simulink model "Prj_1_E"  (R2023a)
settings: Solver=VariableStepAuto  StartTime=0.0  StopTime=600  RelTol=1e-3
model workspace (MAT data in the model file):
  C_0 = 0.015
  M_veh = 1746
  g = 9.8
values from neighbouring files (symbols this model uses):
  A_F = params.FrontalArea_m2_    [Old_Init.m]    (also in init.m; old_script.m)
  C_D = params.Cd    [init.m]
  eta_ess = 0.8    [Old_Init.m]    (also in init.m; old_script.m)
  G_diff = 0.268    [Old_Init.m]    (also in init.m; old_script.m)
  G_elec = 1    [Old_Init.m]    (also in init.m; old_script.m)
  r_wheel = params.WheelRadius_meters_    [init.m]
  rho = params.AirDensity    [init.m]
  SOC_init = 0.5    [Old_Init.m]    (also in init.m; loadVehicleParams.m; old_script.m)
undefined symbols (not defined in the file or in its folder): E_ess_max, eng_map, g_per_hr_to_gal_per_s, m_to_mi, mi_per_hr_to_m_per_s, param, us06
libraries: visionstatistics x1
settings Model: Creator=manuel  LastModifiedBy=Manuel
settings SolverCC: ZeroCrossAlgorithm=Adaptive  AlgebraicLoopSolver=TrustRegion
settings DebuggingCC: MaskedZcDiagnostic=none  IgnoredZcDiagnostic=none  UnconnectedInputMsg=warning  UnconnectedOutputMsg=warning  UnconnectedLineMsg=warning
settings ModelReferenceCC: EnableRefExpFcnMdlSchedulingChecks=on

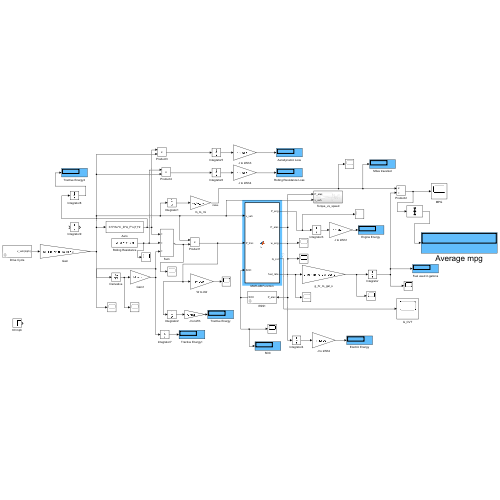
[thumbnail: Simulink's stored preview of the top-level diagram]
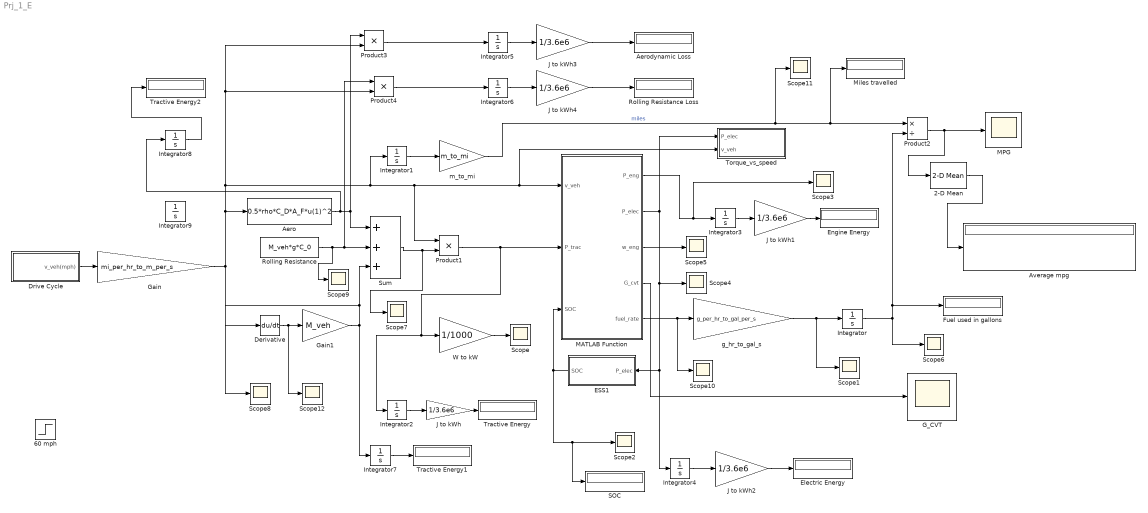
== system Prj_1_E ==
  2-D Mean : visionstatistics/2-D Mean  run=off  reset_popup=None  directionMode=Entire input  dimension=1  treatSBRowAsCol=on  outputLastDataTypeStr=Inherit: Same as accumulator  accumMode=Binary point scaling  accumWordLength=32  accumFracLength=0  accumLastDataTypeStr=fixdt([],32,0)  roiEnable=off  roiType=Rectangles  roiPortion=Entire ROI  roiOutput=Individual statistics for each ROI  roiFlag=off  roundingMode=Floor  overflowMode=off  accumDataTypeStr=fixdt([],32,0)  outputDataTypeStr=Inherit: Same as accumulator  outputMin=[]  outputMax=[]
  60 mph : Step  Before=60  After=60  SampleTime=0
  Aero : Fcn  Expr=0.5*rho*C_D*A_F*u(1)^2
  Aerodynamic Loss : Display
  Average mpg : Display
      settings: Decimation=3
  Derivative : Derivative
  Drive Cycle : Subsystem  mask{schedule=us06}
      mask prompts: schedule "drive schedule"
      mask init:
      | N=length(schedule(:,1))
  ESS1 : Subsystem  mask{E_max=E_ess_max, eta_ess=eta_ess}
      mask prompts: E_max "Maximum energy, J"; eta_ess "round-trip efficiency"
  Electric Energy : Display
  "Engine Energy " : Display
  Fuel used in gallons : Display
  G_CVT : Scope
  Gain : Gain  Gain=mi_per_hr_to_m_per_s
  Gain1 : Gain  Gain=M_veh
  Integrator{,1..9} (10 alike) : Integrator
  J to kWh{,1..4} (5 alike) : Gain  Gain=1/3.6e6
  MATLAB Function : MATLAB Function  TreatAsAtomicUnit=on
  MPG : Scope
  Miles travelled : Display
  Product1 : Product
  Product2 : Product  Inputs=*/
  Product3 : Product
  Product4 : Product
  Rolling Resistance : Constant  Value=M_veh*g*C_0
  Rolling Resistance Loss : Display
  SOC : Display
  Scope{,1..12} (13 alike) : Scope
  Sum : Sum  Inputs=+++
  Torque_vs_speed : Subsystem
  Tractive Energy : Display
  Tractive Energy1 : Display
  Tractive Energy2 : Display
  W to kW : Gain  Gain=1/1000
  g_hr_to_gal_s : Gain  Gain=g_per_hr_to_gal_per_s
  m_to_mi : Gain  Gain=m_to_mi
  wires:
  Aero/1 -> Integrator8/1, Sum/1, Product3/1
  Rolling Resistance/1 -> Scope9/1, Product4/1, Sum/2
  Sum/1 -> Scope7/1, Product1/2
  MATLAB Function/2(P_elec) -> Torque_vs_speed/1(P_elec), Scope4/1, Integrator4/1, ESS1/1(P_elec)
  Gain/1 -> Aero/1, Product1/1, Torque_vs_speed/2(v_veh), MATLAB Function/1(v_veh), Integrator1/1, Product4/2, Product3/2, Derivative/1
  g_hr_to_gal_s/1 -> Integrator/1, Scope1/1
  Integrator1/1 -> m_to_mi/1
  MATLAB Function/1(P_eng) -> Integrator3/1, Scope3/1
  MATLAB Function/3(w_eng) -> Scope5/1
  m_to_mi/1 -> Product2/1, Miles travelled/1, Scope11/1  "miles"
  MATLAB Function/4(G_cvt) -> G_CVT/1
  W to kW/1 -> Scope/1
  Integrator/1 -> Product2/2, Fuel used in gallons/1, Scope6/1
  ESS1/1(SOC) -> SOC/1, Scope2/1, MATLAB Function/3(SOC)
  Product1/1 -> W to kW/1, Integrator2/1, MATLAB Function/2(P_trac)
  Integrator2/1 -> J to kWh/1
  J to kWh/1 -> Tractive Energy/1
  Integrator3/1 -> J to kWh1/1
  J to kWh1/1 -> "Engine Energy "/1
  Integrator4/1 -> J to kWh2/1
  J to kWh2/1 -> Electric Energy/1
  Integrator5/1 -> J to kWh3/1
  J to kWh3/1 -> Aerodynamic Loss/1
  Product3/1 -> Integrator5/1
  Product4/1 -> Integrator6/1
  Integrator6/1 -> J to kWh4/1
  J to kWh4/1 -> Rolling Resistance Loss/1
  Product2/1 -> 2-D Mean/1, MPG/1
  2-D Mean/1 -> Average mpg/1
  MATLAB Function/5(fuel_rate) -> Scope10/1, g_hr_to_gal_s/1
  Drive Cycle/1(v_veh(mph)) -> Gain/1
  Derivative/1 -> Scope12/1, Gain1/1
  Gain1/1 -> Integrator7/1, Scope8/1, Sum/3
  Integrator7/1 -> Tractive Energy1/1
  Integrator8/1 -> Tractive Energy2/1

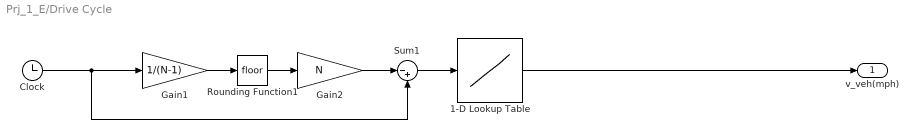
== system Prj_1_E/Drive Cycle ==
  1-D Lookup Table : Lookup_n-D  NumberOfTableDimensions=1  BreakpointsForDimension1=schedule(:,1)  Table=schedule(:,2)  InternalRulePriority=Speed  RndMeth=Simplest
  Clock : Clock
  Gain1 : Gain  Gain=1/(N-1)
  Gain2 : Gain  Gain=N
  Rounding Function1 : Rounding
  Sum1 : Sum  Inputs=|-+
  v_veh(mph) : Outport  VectorParamsAs1DForOutWhenUnconnected=off
  wires:
  Clock/1 -> Gain1/1, Sum1/2
  Sum1/1 -> 1-D Lookup Table/1
  Gain2/1 -> Sum1/1
  Rounding Function1/1 -> Gain2/1
  Gain1/1 -> Rounding Function1/1
  1-D Lookup Table/1 -> v_veh(mph)/1

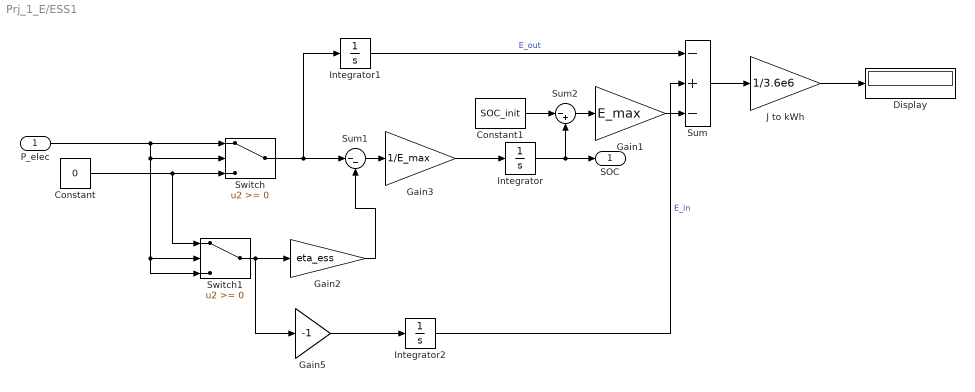
== system Prj_1_E/ESS1 ==
  P_elec : Inport
  Constant : Constant  Value=0
  Constant1 : Constant  Value=SOC_init
  Display : Display
  Gain1 : Gain  Gain=E_max  OutDataTypeStr=fixdt('double', 'DataTypeOverride', 'Off')
  Gain2 : Gain  Gain=eta_ess
  Gain3 : Gain  Gain=1/E_max  OutDataTypeStr=fixdt('double', 'DataTypeOverride', 'Off')
  Gain5 : Gain  Gain=-1  OutDataTypeStr=fixdt('double', 'DataTypeOverride', 'Off')
  Integrator : Integrator  InitialCondition=SOC_init  LimitOutput=on  UpperSaturationLimit=1  LowerSaturationLimit=0
  Integrator1 : Integrator
  Integrator2 : Integrator
  J to kWh : Gain  Gain=1/3.6e6  OutDataTypeStr=fixdt('double', 'DataTypeOverride', 'Off')
  Sum : Sum  Inputs=-+-
  Sum1 : Sum  Inputs=|--
  Sum2 : Sum  Inputs=|-+
  Switch : Switch  OutDataTypeStr=double  SaturateOnIntegerOverflow=off  InputSameDT=off
  Switch1 : Switch  OutDataTypeStr=double  SaturateOnIntegerOverflow=off  InputSameDT=off
  SOC : Outport
  wires:
  P_elec/1 -> Switch1/2, Switch1/3, Switch/2, Switch/1
  Gain3/1 -> Integrator/1
  Gain2/1 -> Sum1/2
  Switch1/1 -> Gain5/1, Gain2/1
  Sum1/1 -> Gain3/1
  Constant/1 -> Switch1/1, Switch/3
  Integrator/1 -> Sum2/2, SOC/1
  Switch/1 -> Integrator1/1, Sum1/1
  Integrator1/1 -> Sum/1  "E_out"
  Integrator2/1 -> Sum/2  "E_in"
  Constant1/1 -> Sum2/1
  Sum2/1 -> Gain1/1
  Gain1/1 -> Sum/3
  Sum/1 -> J to kWh/1
  J to kWh/1 -> Display/1
  Gain5/1 -> Integrator2/1

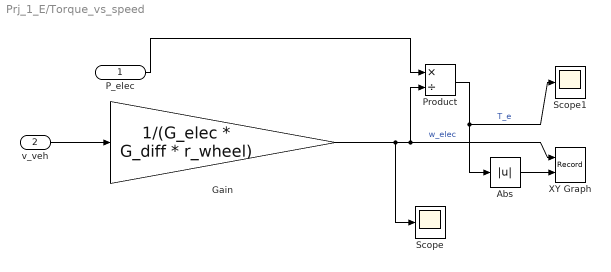
== system Prj_1_E/Torque_vs_speed ==
  P_elec : Inport
  v_veh : Inport  Port=2
  Abs : Abs  SaturateOnIntegerOverflow=off
  Gain : Gain  Gain=1/(G_elec * G_diff * r_wheel)
  Product : Product  Inputs=*/
  Scope : Scope
  Scope1 : Scope
  XY Graph : Record  FileSettingsInternal="{\"entries\":[{\"content\":{\"excelSettings\":{\"content\":{},\"type\":\"Streamout.ExcelSettings\"}},\"type\":\"Streamout.FileSettingStorage\",\"uuid\":\"7cac30b7-4445-42ff-b252-bc9904411e2f\"}],\"packageUris\":[\"http://schema.mathworks.com/mf0/streamout_blocks/R2020a\"],\"version\":\"1.0\"}"  Layout=[1 1]  SignalsInternal="{\"entries\":[{\"content\":{\"signals\":[{\"content\":{\"blockPath\":[\"Prj_1_E/Torque_vs_speed/XY Graph\"],\"dimensions\":[1],\"domain\":\"Prj_1_E/Torque_vs_speed/XY Graph\",\"lineColor\":\"#a2142f\",\"plots\":[1],\"port\":1,\"signalID\":341,\"signalName\":\"w_elec\"},\"type\":\"RecordBlkView.Signal\",\"uuid\":\"f16ed699-5ce4-4a78-9aeb-5aba4233ef7e\"},{\"content\":{\"blockPath\":[\"Prj_1_E/Torque_vs_speed/XY Graph\"],\"dimensions\":[1],\"domain\":\"Prj_1_E/Torque_vs_speed/XY Graph\",\"lineColor\":\"#139fff\",\"plots\":[1],\"port\":2,\"signalID\":344,\"signalName\":\"Abs\"},\"type\":\"RecordBlkView.Signal\",\"uuid\":\"74b02491-6fa4-4c43-b90e-f85759798827\"}]},\"type\":\"RecordBlkView.InputSignals\",\"uuid\":\"1f05e0d2-8816-4d0d-9217-ea4bf3e9380e\"}],\"packageUris\":[\"http://schema.mathworks.com/mf0/streamout_blocks/R2020a\"],\"version\":\"1.0\"}"  VisualizationBindings="{\"xyplotplugin\":{\"info\":[{\"series\":[{\"bindingParametersList\":[{\"parameter\":\"X-Axis\",\"signalID\":341,\"signalName\":\"w_elec\"},{\"parameter\":\"Y-Axis\",\"signalID\":344,\"signalName\":\"Abs\"}],\"seriesID\":13028}],\"subplotID\":1}]}}"  CompatibilityTag=XY  st=-1
  wires:
  Abs/1 -> XY Graph/2
  Gain/1 -> Scope/1, Product/2, XY Graph/1  "w_elec"
  v_veh/1 -> Gain/1
  Product/1 -> Abs/1, Scope1/1  "T_e"
  P_elec/1 -> Product/1

== matlab function Prj_1_E/MATLAB Function ==
  data: v_veh input; P_eng output; P_trac input; SOC input; P_elec output; w_eng output; G_cvt output; fuel_rate output; param parameter; eng_map parameter
function [P_eng, P_elec, w_eng, G_cvt, fuel_rate] = fcn(v_veh, P_trac, SOC, param, eng_map)
%#codegen
%inputs:
    % v_veh, m/s
    % P_trac, W
    % SOC
    % param, structure of parameters
    % eng_map

% outputs:
    %   P_gen, P_elec in W
    %   w_eng, rpm
    %   G_cvt (cvt ratio)
    %   Fuel rate, g/hr

v_veh_min = param.v_veh_min;    % minimum vehicle speed for engine to stay engaged, in m/s
P_eng_min = param.P_eng_min;    % minimum engine power in W
P_eng_max = param.P_eng_max ;   % maximum engine power
G_cvt_min = param.G_cvt_min;    % minimum cvt  ratio
G_diff = param.G_diff;          % differential gear ratio
r_wheel = param.r_wheel;        % wheel radius in m

%All Electric mode
if (v_veh < v_veh_min)  % disengage clutch, idle, engine, electric launch
    P_elec = P_trac;
    P_eng = 0;
    fuel_rate = 450; % g/hr;
    w_eng = 1000; % rpm
    G_cvt = G_cvt_min;
    return  
end

% if here, v_veh > v_veh_min
if(P_trac < P_eng_min)   % clutch engaged but no fuel
   P_elec = P_trac;
   fuel_rate = 0;
   P_eng = 0;
   w_eng =  1000; % rpm
   w_eng_SI = w_eng * 2 * pi / 60; % rad/s
   % set G_cvt so engine speed is 1000 rpm
   G_cvt = v_veh/G_diff/w_eng_SI/r_wheel;
   return     
end

%It never reaches this point in us06
if(P_trac > P_eng_max) % high-speed boost
   P_elec = P_trac - P_eng_max;
   P_eng = P_eng_max;
   bsfc = interp1(eng_map(:,2), eng_map(:,3), P_eng/1000);
   fuel_rate = bsfc*P_eng/1000; % g/hr
   w_eng = interp1(eng_map(:,2), eng_map(:,1), P_eng/1000);
   w_eng_SI = w_eng * 2 * pi / 60; % convert to rad/s
   G_cvt =  v_veh/r_wheel/G_diff/w_eng_SI; % required CVT ratio
   return   
end

% if here, v_veh > v_veh_min and P_eng_min < P_trac < P_eng_max
% try to get SOC back to 0.5

P_elec = 4000*sign(SOC - 0.5); 
P_eng = P_trac - P_elec;

if(P_eng < P_eng_min) 
   % clutch engaged, but no fuel
   P_eng = 0;
   P_elec = P_trac;
   fuel_rate = 0;
   w_eng = 1000;
   w_eng_SI = w_eng * 2 * pi / 60; % om rad/s
   % set G_cvt so engine speed is 1000 rpm
   G_cvt = v_veh/G_diff/w_eng_SI/r_wheel;
   return
end

if(P_eng > P_eng_max)
    P_eng = P_eng_max;
    P_elec = P_trac - P_eng_max;
end

bsfc = interp1(eng_map(:,2), eng_map(:,3), P_eng/1000);
fuel_rate = bsfc*P_eng/1000; % g/hr

w_eng = interp1(eng_map(:,2), eng_map(:,1), P_eng/1000);%How this work?
w_eng_SI = w_eng* pi / 30;  % convert to rad/s
G_cvt =  v_veh/r_wheel/G_diff/w_eng_SI;

if (G_cvt < G_cvt_min) % disengage clutch, idle engine
   P_eng = 0;
   P_elec = P_trac;
   G_cvt = G_cvt_min;
   fuel_rate = 450;
   w_eng = 1000; % rpm
 end
